simulink model "GA_test"  (R2022a)
settings: Solver=VariableStepAuto  StartTime=0.0  StopTime=0.2  RelTol=1e-3
values from neighbouring files (symbols this model uses):
  d0 = 1e-09    [ga_5.mat]    (also in ga_6.mat; ga_ok_1.mat; ga_ok_10.mat; ga_ok_2.mat)
  fs = 30000    [ga_5.mat]    (also in ga_6.mat; ga_ok_1.mat; ga_ok_10.mat; ga_ok_2.mat)
  g = 0.0011    [ga_5.mat]    (also in ga_6.mat; ga_ok_1.mat; ga_ok_10.mat; ga_ok_2.mat)
  Ga = 1.2e-09    [ga_5.mat]    (also in ga_6.mat; ga_ok_1.mat; ga_ok_10.mat; ga_ok_2.mat)
  Gc = 1000000000    [ga_5.mat]    (also in ga_6.mat; ga_ok_1.mat; ga_ok_10.mat; ga_ok_2.mat)
  Gv = 15    [ga_5.mat]    (also in ga_6.mat; ga_ok_1.mat; ga_ok_10.mat; ga_ok_2.mat)
  k = 16500000000    [ga_5.mat]    (also in ga_6.mat; ga_ok_1.mat; ga_ok_10.mat; ga_ok_2.mat)
  R = conv(Hr, [parms(1) parms(2)])    [controller_test.m]    (also in controller_test_ok_10.m; controller_test_ok_3.m; controller_test_ok_6.m; controller_test_ok_7.m)
  S = conv(Hs, [1 parms(3) parms(4)])    [controller_test.m]    (also in controller_test_ok_10.m; controller_test_ok_3.m; controller_test_ok_6.m; controller_test_ok_7.m)
  vb = 1.025    [ga_5.mat]    (also in ga_6.mat; ga_ok_1.mat; ga_ok_10.mat; ga_ok_2.mat)
  wa = 120000    [ga_5.mat]    (also in ga_6.mat; ga_ok_1.mat; ga_ok_10.mat; ga_ok_2.mat)
  wc = 13000    [ga_5.mat]    (also in ga_6.mat; ga_ok_1.mat; ga_ok_10.mat; ga_ok_2.mat)
  wv = 4000    [ga_5.mat]    (also in ga_6.mat; ga_ok_1.mat; ga_ok_10.mat; ga_ok_2.mat)
  zeta = 0.9    [ga_5.mat]    (also in ga_6.mat; ga_ok_1.mat; ga_ok_10.mat; ga_ok_2.mat)
libraries: simulink x1
settings Model: Creator=doamarar  LastModifiedBy=doamarar
settings DataIOCC: InspectSignalLogs=on  ReturnWorkspaceOutputs=off

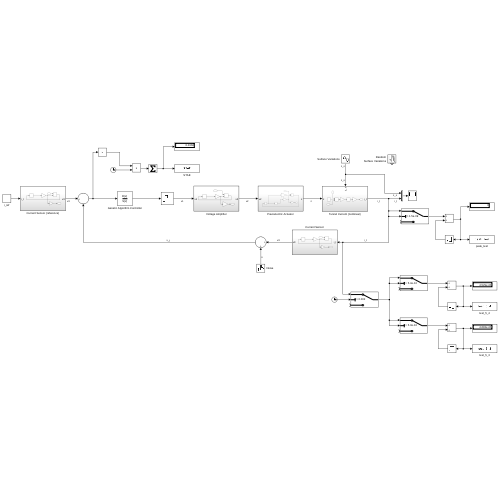
[thumbnail: Simulink's stored preview of the top-level diagram]
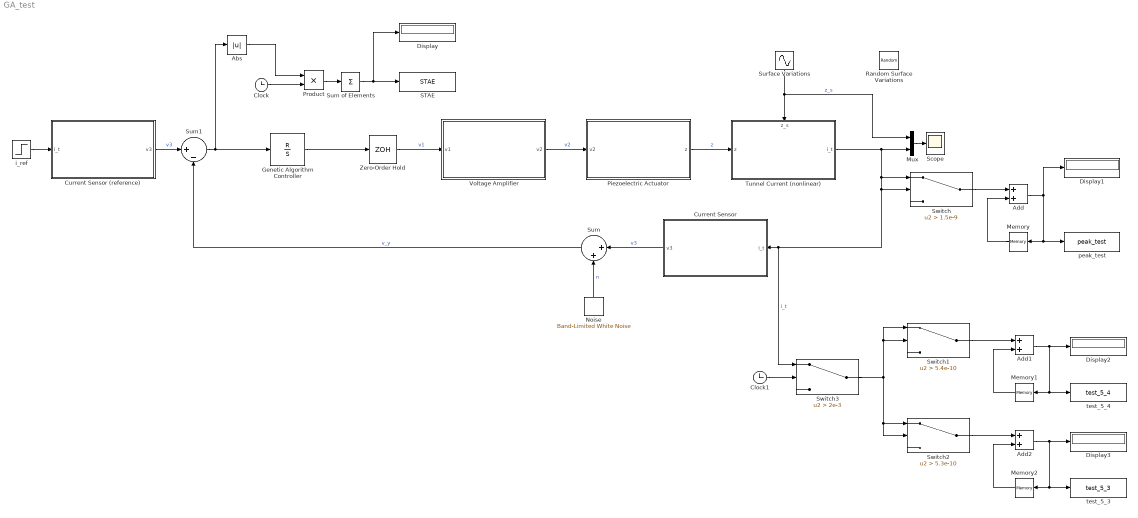
== system GA_test ==
  Abs : Abs  SaturateOnIntegerOverflow=off
  Add : Sum
  Add1 : Sum
  Add2 : Sum
  Clock : Clock
  Clock1 : Clock
  Current Sensor : Subsystem
  Current Sensor (reference) : Subsystem
  Display{,1..3} (4 alike) : Display
  Genetic Algorithm Controller : DiscreteFilter  Numerator=R  Denominator=S  SampleTime=1/fs
  Memory : Memory
  Memory1 : Memory
  Memory2 : Memory
  Mux : Mux  Inputs=2
  Noise : simulink/Sources/Band-Limited White Noise  Cov=[0.000000001]  Ts=1/fs  seed=[23341]
  Piezoelectric Actuator : Subsystem
  Product : Product
  Random Surface Variations : RandomNumber  Variance=2*10^-25  SampleTime=0.0000333333
  STAE : ToWorkspace  VariableName=STAE  SampleTime=-1
  Scope : Scope
  Sum : Sum  Inputs=|++
  Sum of Elements : Sum  Inputs=+
  Sum1 : Sum  Inputs=|+-
  Surface Variations : Sin  Amplitude=5*10^-11  Frequency=600  SampleTime=1/fs
  Switch : Switch  Criteria=u2 > Threshold  Threshold=1.5e-9  SaturateOnIntegerOverflow=off  InputSameDT=off
  Switch1 : Switch  Criteria=u2 > Threshold  Threshold=5.4e-10  SaturateOnIntegerOverflow=off  InputSameDT=off
  Switch2 : Switch  Criteria=u2 > Threshold  Threshold=5.3e-10  SaturateOnIntegerOverflow=off  InputSameDT=off
  Switch3 : Switch  Criteria=u2 > Threshold  Threshold=2e-3  SaturateOnIntegerOverflow=off  InputSameDT=off
  Tunnel Current (nonlinear) : Subsystem
      settings: PortSchema="{\"entries\":[{\"content\":{\"sides\":[{\"content\":{\"connectorIds\":[\"In1\"]},\"type\":\"ConnectorPlacement.EquallySpacedRectSide\",\"uuid\":\"147d123d-45a5-4220-b41f-835da98fb0cd\"},{\"content\":{\"connectorIds\":[\"Out1\"],\"side\":\"RIGHT\"},\"type\":\"ConnectorPlacement.EquallySpacedRectSide\",\"uuid\":\"1a05abba-b8fc-4d61-92c8-15761dd3dd6b\"},{\"content\":{\"connectorIds\":[\"In2\"],\"side\":\"TOP\"},\"type\":\"ConnectorPlacement.EquallySpacedRectSide\",\"uuid\":\"bc9d4ee1-4dd7-4150-9ece-b291902d4347\"}]},\"type\":\"ConnectorPlacement.EquallySpacedConnector\",\"uuid\":\"916abd9f-079e-4be3-a864-fdb35439c6f4\"}],\"packageUris\":[\"http://schema.mathworks.com/mf0/Connector/R2020b\"],\"version\":\"1.0\"}"
  Voltage Amplifier : Subsystem
  Zero-Order Hold : ZeroOrderHold  SampleTime=1/fs
  i_ref : Step  Time=0  After=0.5*10^-9  SampleTime=1/fs
  peak_test : ToWorkspace  VariableName=peak_test  SampleTime=-1
  test_5_3 : ToWorkspace  VariableName=test_5_3  SampleTime=-1
  test_5_4 : ToWorkspace  VariableName=test_5_4  SampleTime=-1
  wires:
  i_ref/1 -> Current Sensor (reference)/1(i_t)
  Voltage Amplifier/1(v2) -> Piezoelectric Actuator/1(v2)  "v2"
  Piezoelectric Actuator/1(z) -> Tunnel Current (nonlinear)/1(z)  "z"
  Surface Variations/1 -> Mux/1, Tunnel Current (nonlinear)/2(z_s)  "z_s"
  Current Sensor/1(v3) -> Sum/1  "v3"
  Noise/1 -> Sum/2  "n"
  Sum/1 -> Sum1/2  "v_y"
  Zero-Order Hold/1 -> Voltage Amplifier/1(v1)  "v1"
  Current Sensor (reference)/1(v3) -> Sum1/1  "v3"
  Mux/1 -> Scope/1
  Clock/1 -> Product/2
  Sum of Elements/1 -> Display/1, STAE/1
  Product/1 -> Sum of Elements/1
  Abs/1 -> Product/1
  Sum1/1 -> Abs/1, Genetic Algorithm Controller/1
  Switch/1 -> Add/1
  Add/1 -> Memory/1, peak_test/1, Display1/1
  Memory/1 -> Add/2
  Memory1/1 -> Add1/2
  Add1/1 -> Display2/1, test_5_4/1, Memory1/1
  Switch1/1 -> Add1/1
  Tunnel Current (nonlinear)/1(i_t) -> Mux/2, Switch3/1, Current Sensor/1(i_t), Switch/2, Switch/1  "i_t"
  Switch2/1 -> Add2/1
  Memory2/1 -> Add2/2
  Add2/1 -> Display3/1, test_5_3/1, Memory2/1
  Clock1/1 -> Switch3/2
  Switch3/1 -> Switch2/2, Switch2/1, Switch1/2, Switch1/1
  Genetic Algorithm Controller/1 -> Zero-Order Hold/1

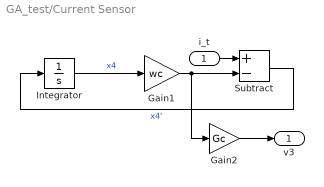
== system GA_test/Current Sensor ==
  i_t : Inport
  Gain1 : Gain  Gain=wc
  Gain2 : Gain  Gain=Gc
  Integrator : Integrator
  Subtract : Sum  Inputs=+-
  v3 : Outport
  wires:
  Gain2/1 -> v3/1
  Integrator/1 -> Gain1/1  "x4"
  Gain1/1 -> Gain2/1, Subtract/2
  i_t/1 -> Subtract/1
  Subtract/1 -> Integrator/1  "x4'"

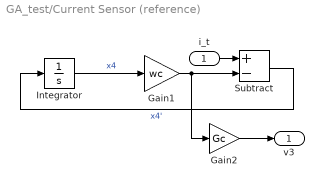
== system GA_test/Current Sensor (reference) ==
  i_t : Inport
  Gain1 : Gain  Gain=wc
  Gain2 : Gain  Gain=Gc
  Integrator : Integrator
  Subtract : Sum  Inputs=+-
  v3 : Outport
  wires:
  Gain2/1 -> v3/1
  Integrator/1 -> Gain1/1  "x4"
  Gain1/1 -> Gain2/1, Subtract/2
  i_t/1 -> Subtract/1
  Subtract/1 -> Integrator/1  "x4'"

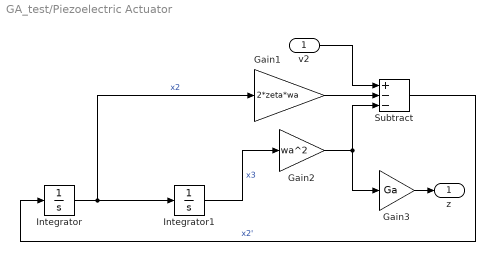
== system GA_test/Piezoelectric Actuator ==
  v2 : Inport
  Gain1 : Gain  Gain=2*zeta*wa
  Gain2 : Gain  Gain=wa^2
  Gain3 : Gain  Gain=Ga
  Integrator : Integrator
  Integrator1 : Integrator
  Subtract : Sum  Inputs=+--
  z : Outport
  wires:
  Subtract/1 -> Integrator/1  "x2'"
  Gain1/1 -> Subtract/2
  v2/1 -> Subtract/1
  Gain2/1 -> Gain3/1, Subtract/3
  Integrator/1 -> Gain1/1, Integrator1/1  "x2"
  Gain3/1 -> z/1
  Integrator1/1 -> Gain2/1  "x3"

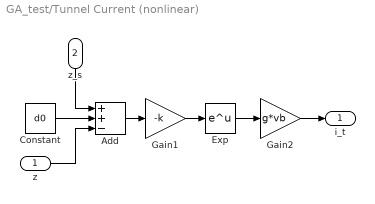
== system GA_test/Tunnel Current (nonlinear) ==
  z : Inport
  z_s : Inport  Port=2
  Add : Sum  Inputs=++-
  Constant : Constant  Value=d0
  Exp : Math
  Gain1 : Gain  Gain=-k
  Gain2 : Gain  Gain=g*vb
  i_t : Outport
  wires:
  Add/1 -> Gain1/1
  z_s/1 -> Add/1
  z/1 -> Add/3
  Gain1/1 -> Exp/1
  Exp/1 -> Gain2/1
  Gain2/1 -> i_t/1
  Constant/1 -> Add/2

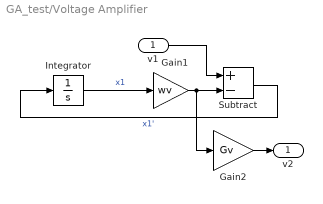
== system GA_test/Voltage Amplifier ==
  v1 : Inport
  Gain1 : Gain  Gain=wv
  Gain2 : Gain  Gain=Gv
  Integrator : Integrator
  Subtract : Sum  Inputs=+-
  v2 : Outport
  wires:
  Integrator/1 -> Gain1/1  "x1"
  Subtract/1 -> Integrator/1  "x1'"
  Gain1/1 -> Gain2/1, Subtract/2
  Gain2/1 -> v2/1
  v1/1 -> Subtract/1
